simulink model "Dynamics"  (R2021a)
settings: Solver=FixedStepAuto  StartTime=0.0  StopTime=1000.0  FixedStep=0.1  RelTol=1e-3
values from neighbouring files (symbols this model uses):
  stateinitial = [x0;y0;z0;xdot0;ydot0;zdot0;q0123_0;p0;q0;r0]    [main.m]
  Ts = 0.1    [myStateTransitionFcn.m]
undefined symbols (not defined in the file or in its folder): m_noise, p_noise
libraries: simulink x2, sharedtransform x2, sharedTrackingLibrary x1
settings Model: Creator=panch  LastModifiedBy=panch

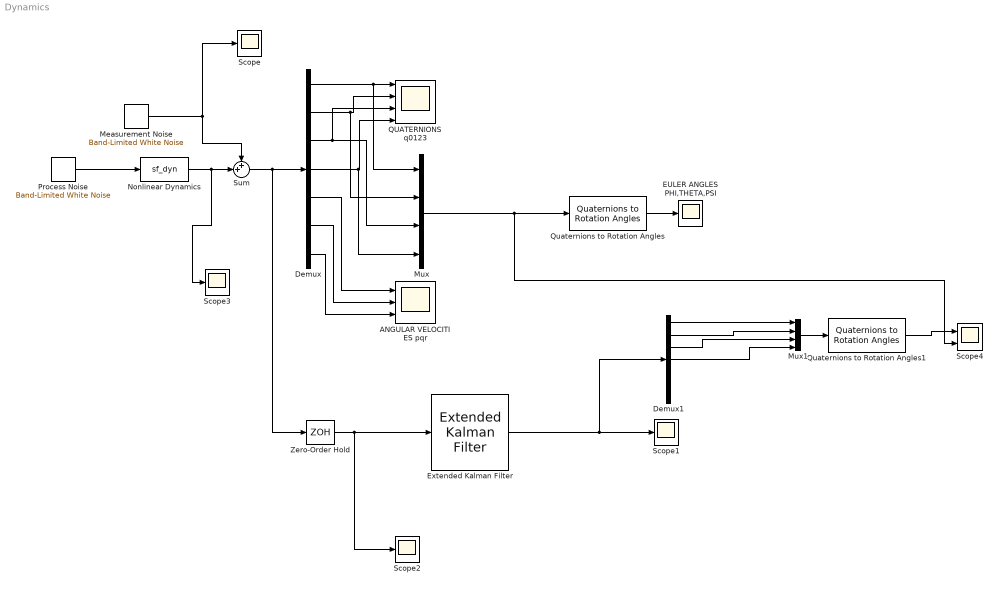
== system Dynamics ==
  ANGULAR VELOCITIES pqr : Scope  NumInputPorts=3
  Demux : Demux  Outputs=7
  Demux1 : Demux  Outputs=7
  EULER ANGLES PHI,THETA,PSI : Scope
  Extended Kalman Filter : sharedTrackingLibrary/Extended Kalman Filter  StateTransitionFcn=myStateTransitionFcn  HasStateTransitionJacobianFcn=off  HasAdditiveProcessNoise=Additive  ProcessNoise=diag(p_noise)  HasTimeVaryingProcessNoise=off  HasStateTransitionFcnExtraArgument=0  InitialState=stateinitial+0.5  InitialStateCovariance=1e-16  MeasurementFcn1=myMeasurementFcn  HasMeasurementJacobianFcn1=off  HasMeasurementEnablePort1=off  HasAdditiveMeasurementNoise1=Additive  MeasurementNoise1=diag(m_noise)  HasTimeVaryingMeasurementNoise1=off  HasMeasurementFcnExtraArgument1=0  MeasurementFcn2=myMeasurementFcn  HasMeasurementJacobianFcn2=off  HasMeasurementEnablePort2=off  HasAdditiveMeasurementNoise2=Additive  MeasurementNoise2=1  HasTimeVaryingMeasurementNoise2=off  HasMeasurementFcnExtraArgument2=0  MeasurementFcn3=myMeasurementFcn  HasMeasurementJacobianFcn3=off  HasMeasurementEnablePort3=off  HasAdditiveMeasurementNoise3=Additive  MeasurementNoise3=1  HasTimeVaryingMeasurementNoise3=off  HasMeasurementFcnExtraArgument3=0  MeasurementFcn4=myMeasurementFcn  HasMeasurementJacobianFcn4=off  HasMeasurementEnablePort4=off  HasAdditiveMeasurementNoise4=Additive  MeasurementNoise4=1  HasTimeVaryingMeasurementNoise4=off  HasMeasurementFcnExtraArgument4=0  MeasurementFcn5=myMeasurementFcn  HasMeasurementJacobianFcn5=off  HasMeasurementEnablePort5=off  HasAdditiveMeasurementNoise5=Additive  MeasurementNoise5=1  HasTimeVaryingMeasurementNoise5=off  HasMeasurementFcnExtraArgument5=0  EnableMultirate=off  StateTransitionFcnSampleTime=1  MeasurementFcn1SampleTime=1  MeasurementFcn2SampleTime=1  MeasurementFcn3SampleTime=1  MeasurementFcn4SampleTime=1  MeasurementFcn5SampleTime=1  UseCurrentEstimator=on  OutputStateCovariance=off  DataType=double  SampleTime=Ts  NumberOfMeasurements=1
      settings: SourceProductBaseCode=CT,DR,TF,ID,LP,NV,AR,RO,RR,UV,VE
  Measurement Noise : simulink/Sources/Band-Limited White Noise  Cov=m_noise*Ts  Ts=Ts  seed=[12347]  VectorParams1D=off
  Mux : Mux
  Mux1 : Mux
  Nonlinear Dynamics : S-Function  FunctionName=sf_dyn  SFunctionDeploymentMode=off  EnableBusSupport=off
  Process Noise : simulink/Sources/Band-Limited White Noise  Cov=p_noise*Ts  Ts=Ts  seed=[23341]  VectorParams1D=off
  QUATERNIONS q0123 : Scope  NumInputPorts=4
  Quaternions to Rotation Angles : sharedtransform/Quaternions to Rotation Angles  rotationOrder=ZYX  aMode=aMode
      settings: SourceProductBaseCode=AE,PW,DR,MT,UV,VE
  Quaternions to Rotation Angles1 : sharedtransform/Quaternions to Rotation Angles  rotationOrder=ZYX  aMode=aMode
      settings: SourceProductBaseCode=AE,PW,DR,MT,UV,VE
  Scope{,1..3} (4 alike) : Scope
  Scope4 : Scope  NumInputPorts=2
  Sum : Sum  Inputs=++|
  Zero-Order Hold : ZeroOrderHold  SampleTime=Ts
  wires:
  Sum/1 -> Zero-Order Hold/1, Demux/1
  Quaternions to Rotation Angles/1 -> EULER ANGLES PHI,THETA,PSI/1
  Zero-Order Hold/1 -> Scope2/1, Extended Kalman Filter/1
  Demux/7 -> ANGULAR VELOCITIES pqr/3
  Demux/4 -> Mux/4, QUATERNIONS q0123/4
  Extended Kalman Filter/1 -> Demux1/1, Scope1/1
  Demux/5 -> ANGULAR VELOCITIES pqr/1
  Demux/6 -> ANGULAR VELOCITIES pqr/2
  Mux/1 -> Scope4/2, Quaternions to Rotation Angles/1
  Process Noise/1 -> Nonlinear Dynamics/1
  Measurement Noise/1 -> Scope/1, Sum/1
  Demux/3 -> Mux/3, QUATERNIONS q0123/3
  Demux/2 -> Mux/2, QUATERNIONS q0123/2
  Demux/1 -> Mux/1, QUATERNIONS q0123/1
  Nonlinear Dynamics/1 -> Sum/2, Scope3/1
  Mux1/1 -> Quaternions to Rotation Angles1/1
  Demux1/1 -> Mux1/1
  Demux1/2 -> Mux1/2
  Demux1/3 -> Mux1/3
  Demux1/4 -> Mux1/4
  Quaternions to Rotation Angles1/1 -> Scope4/1
